simulink model "zad1"  (R2018a)
settings: Solver=VariableStepAuto  StartTime=0.0  StopTime=1000  RelTol=1e-3
values from neighbouring files (symbols this model uses):
  alfa1 = 0.15    [MODI_Projekt1.m]
  alfa2 = -0.16    [MODI_Projekt1.m]
  alfa3 = 0.25    [MODI_Projekt1.m]
  alfa4 = 0.43    [MODI_Projekt1.m]
  K = 2    [MODI_Projekt1.m]
  T1 = 9    [MODI_Projekt1.m]
  T2 = 6    [MODI_Projekt1.m]
  u_p = 0.5    [MODI_Projekt1.m]
  x1_p = 0    [MODI_Projekt1.m]
  x2_p = 0    [MODI_Projekt1.m]
settings Model: Creator=gajee  LastModifiedBy=gajee

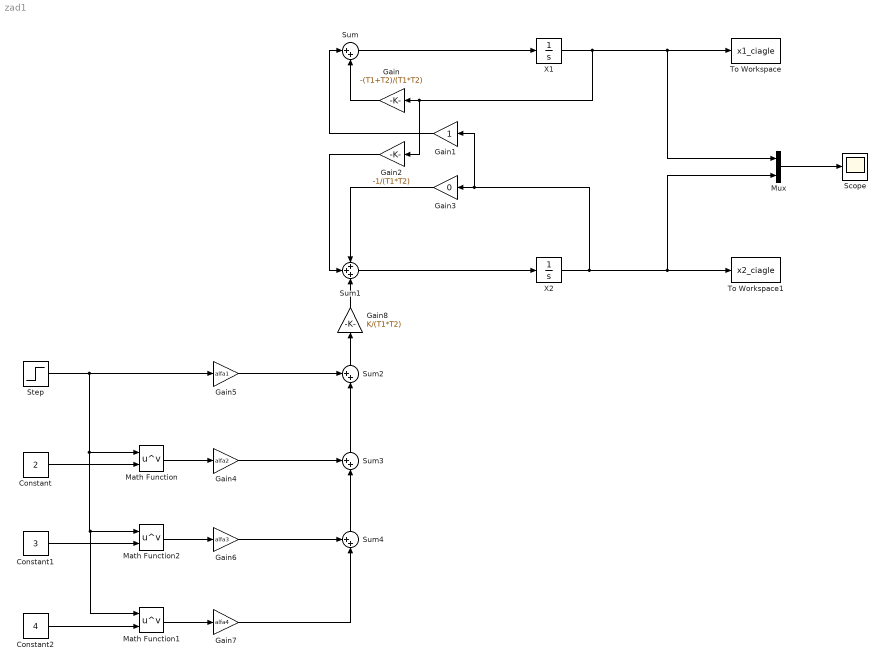
== system zad1 ==
  Constant : Constant  Value=2
  Constant1 : Constant  Value=3
  Constant2 : Constant  Value=4
  Gain : Gain  Gain=-(T1+T2)/(T1*T2)
  Gain1 : Gain
  Gain2 : Gain  Gain=-1/(T1*T2)
  Gain3 : Gain  Gain=0
  Gain4 : Gain  Gain=alfa2
  Gain5 : Gain  Gain=alfa1
  Gain6 : Gain  Gain=alfa3
  Gain7 : Gain  Gain=alfa4
  Gain8 : Gain  Gain=K/(T1*T2)
  Math Function : Math  Operator=pow  SaturateOnIntegerOverflow=on
  Math Function1 : Math  Operator=pow  SaturateOnIntegerOverflow=on
  Math Function2 : Math  Operator=pow  SaturateOnIntegerOverflow=on
  Mux : Mux  Inputs=2
  Scope : Scope
  Step : Step  Before=u_p  After=u  SampleTime=0
  Sum : Sum  Inputs=|++
  Sum1 : Sum  Inputs=+++
  Sum2 : Sum  Inputs=++|
  Sum3 : Sum  Inputs=++|
  Sum4 : Sum  Inputs=++|
  To Workspace : ToWorkspace  VariableName=x1_ciagle  SaveFormat=Structure With Time  SampleTime=-1
  To Workspace1 : ToWorkspace  VariableName=x2_ciagle  SaveFormat=Structure With Time  SampleTime=-1
  X1 : Integrator  InitialCondition=x1_p
  X2 : Integrator  InitialCondition=x2_p
  wires:
  X1/1 -> Gain2/1, Gain/1, To Workspace/1, Mux/1
  X2/1 -> Gain1/1, Gain3/1, To Workspace1/1, Mux/2
  Gain1/1 -> Sum/1
  Gain/1 -> Sum/2
  Sum/1 -> X1/1
  Gain2/1 -> Sum1/2
  Gain3/1 -> Sum1/1
  Sum1/1 -> X2/1
  Gain7/1 -> Sum4/2
  Math Function1/1 -> Gain7/1
  Math Function2/1 -> Gain6/1
  Math Function/1 -> Gain4/1
  Gain4/1 -> Sum3/1
  Sum4/1 -> Sum3/2
  Sum3/1 -> Sum2/2
  Gain5/1 -> Sum2/1
  Step/1 -> Math Function/1, Math Function1/1, Math Function2/1, Gain5/1
  Constant/1 -> Math Function/2
  Constant1/1 -> Math Function2/2
  Constant2/1 -> Math Function1/2
  Gain6/1 -> Sum4/1
  Mux/1 -> Scope/1
  Gain8/1 -> Sum1/3
  Sum2/1 -> Gain8/1
